simulink model "sample_model"  (R2023a)
settings: Solver=ode5  StartTime=0.0  StopTime=Inf  FixedStep=0.0001  RelTol=1e-3
PostLoadFcn:
  | , if any(exist('dsrtsu_mdlpostloadfcn', 'file') ~= 0), dsrtsu_mdlpostloadfcn('Execute', bdroot); end,
InitFcn:
  | , if any(exist('rtifpga_mdlclblib', 'file') ~= 0), rtifpga_mdlclblib('Init', bdroot); end,
values from neighbouring files (symbols this model uses):
  alpha = 0    [freq_sweep.m]    (also in freq_sweep_continous.m; single_test.m)
  k_harmonics = 7    [freq_sweep.m]    (also in freq_sweep_continous.m; single_test.m)
libraries: rti1202lib_adc_class1 x3, rti1202lib_dac_class1 x2, simulink x2, rti1202lib_base x1
(part 1 of 2)
Description:
  | Standard RTI1202 template.
  | Supported MATLAB version:  R2023a.
settings Model: Tag=RTI1202  DSRTSU_INTERNAL_RTI_VER=620  DSRTSU_INTERNAL_RTI_TYPE=rti1202  RTICANMMDATA=struct('GeneralSetupData',struct('modelroot','C:\Users\VM-User\Desktop\MigrationScripts','generalsettings',struct('filesettings',struct('destfolder',struct('Name','RTICANMM_FILES','Check',1),'buildfolder',struct('Name','.','Check',1),'AbsDestfolder',struct('Name','C:\Users\VM-User\Desktop\MigrationScripts\RTICANMM_FILES'),'AbsBuildfolder',struct('Name','C:\Users\VM-User\Desktop\MigrationScripts'))),'options',struct('addpaths',1,'rmpaths',1,'addtrcexclusion',true,'cannavigator',struct('checkmonitoring',0),'show_usrtrc',0,'use_usrtrc',0),'advanced',struct('options',ones(1,100)),'MPSetup',{{}},'RTI',struct('Type','RTI1202','Ver','7.17','Date','02-Nov-2021'),'modelname','','block','untitled'))  DSRTSU_INTERNAL_RTIFPGA=200  DSRTSU_INTERNAL_RTISTBM_VER=23.1  Creator=akb110  LastModifiedBy=dionl
settings SolverCC: AlgebraicLoopSolver=TrustRegion
settings DataIOCC: ReturnWorkspaceOutputs=off
settings OptimizationCC: BlockReduction=off  OptimizeBlockIOStorage=off  BufferReuse=off  ReuseModelBlockBuffer=off  GlobalBufferReuse=off  ExpressionFolding=off  LocalBlockOutputs=off  OptimizeDataStoreBuffers=off  BusAssignmentInplaceUpdate=off
settings DebuggingCC: UnconnectedInputMsg=warning  UnconnectedOutputMsg=warning  UnconnectedLineMsg=warning  PregeneratedLibrarySubsystemCodeDiagnostic=none  ArithmeticOperatorsInVariantConditions=warning
settings HardwareCC: ProdBitPerPointer=32  ProdBitPerSizeT=32  ProdBitPerPtrDiffT=32  ProdLargestAtomicInteger=Integer  ProdEndianess=BigEndian  ProdWordSize=32  ProdLongLongMode=on  ProdHWDeviceType=Custom Processor->Custom  TargetIntDivRoundTo=Zero  TargetEndianess=BigEndian  TargetHWDeviceType=Custom Processor->Custom
settings ModelReferenceCC: EnableRefExpFcnMdlSchedulingChecks=on  EnableParallelModelReferenceBuilds=on  ParallelModelReferenceMATLABWorkerInit=Load Top Model
settings SFSimCC: SimUseLocalCustomCode=off  MATLABDynamicMemAlloc=off  CustomCodeUndefinedFunction=UseInterfaceOnly
settings RTWCC: Description=dSPACE DS1202 Hardware Platform  SystemTargetFile=rti1202.tlc  MakeCommand=make_rti  TemplateMakefile=rti1202.tmf  RTWUseLocalCustomCode=off  DLArmComputeVersion=19.05
settings CodeAppCC: StateflowObjectComments=on
settings STFCustomTargetCC: TargetLangStandard=C89/C90 (ANSI)  ParMdlRefBuildCompliant=on  ConcurrentExecutionCompliant=off  GRTInterface=off  UseToolchainInfoCompliant=off  SystemTargetFile=rti1202.tlc
settings GRTTargetCC: TargetLangStandard=C89/C90 (ANSI)  CompOptLevelCompliant=off  ConcurrentExecutionCompliant=off  CombineOutputUpdateFcns=off  MatFileLogging=off  CPPClassGenCompliant=off  UseToolchainInfoCompliant=off
settings ConfigComp: CovMetricSettings=dswe

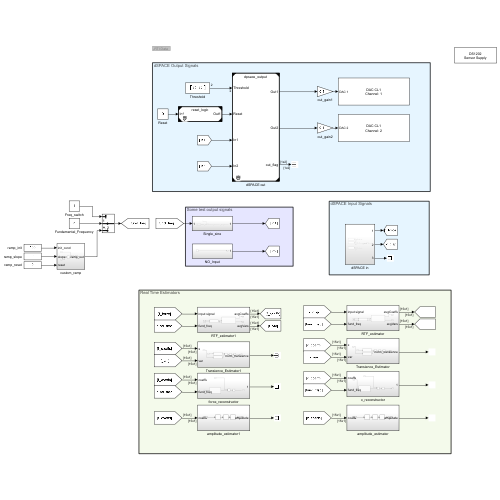
[thumbnail: Simulink's stored preview of the top-level diagram]
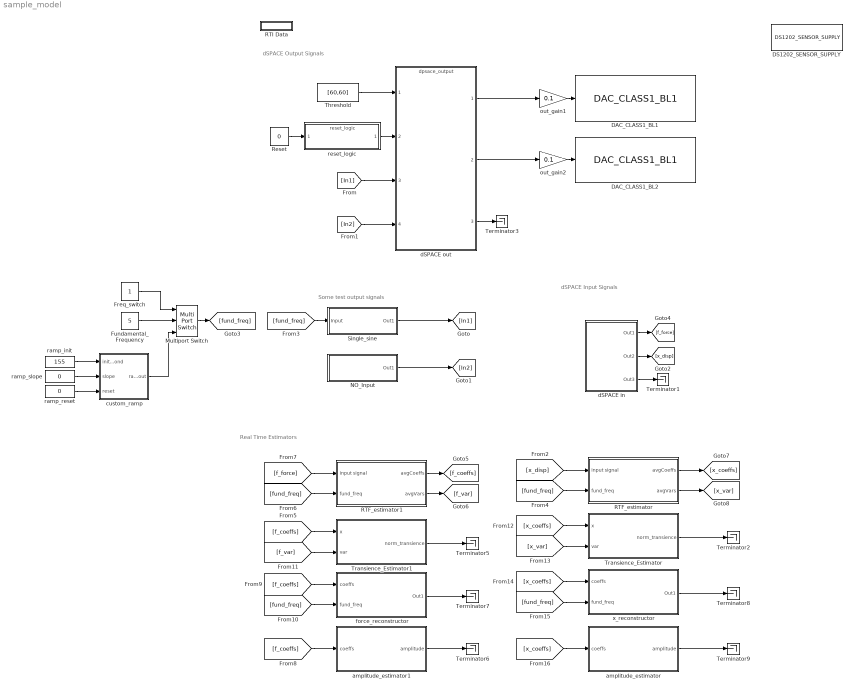
== system sample_model ==
  note: Real Time Estimators
  note: dSPACE Input Signals
  note: dSPACE Output Signals
  note: Some test output signals
  DAC_CLASS1_BL1 : rti1202lib_dac_class1/DAC_CLASS1_BL1  DSProperties=struct('RTI',struct('Version',uint32(2),'BlockType',struct('isSLSource',uint8(0),'isSLSink',uint8(1),'isHWSource',uint8(0),'isHWSink',uint8(1),'isSetup',uint8(0),'isInline',uint8(1),'isNonInline',uint8(0),'isInterrupt',uint8(0),'isChannelwise',uint8(1)),'IOBoardType',{{'DS120X','STD','DACC1'}},'UnitType','DAC','Identifier','DAC','DialogType','ML','BlockSet','NONE','SlaveProcessor','NONE'))  RTIBlockInterface=struct('InputPortsActive',1,'InputPortsWidth',int32(1),'InputPortsDataType',{{'SS_DOUBLE'}},'InputPortsName',{{['DAC 1']}},'DialogFcn','rti120xstddacc1dacgui','InitLevel',3,'IconTransparency','on','BlockDisplay',{{['DAC CL1\nChannel: 1'],'center'}},'BlockName',struct('Token',{{'DAC_CLASS1_BL1'}}))  RTIBlockParameters=struct('ChannelNo',{{1,'OFF',[]}},'ChannelNumOf',{{1,'OFF',[]}},'InitialValue1',{{0,'OFF',[-10 10]}},'InitialValue2',{{0,'OFF',[-10 10]}},'InitialValue3',{{0,'OFF',[-10 10]}},'InitialValue4',{{0,'OFF',[-10 10]}},'InitialValue5',{{0,'OFF',[-10 10]}},'InitialValue6',{{0,'OFF',[-10 10]}},'InitialValue7',{{0,'OFF',[-10 10]}},'InitialValue8',{{0,'OFF',[-10 10]}},'InitialValue9',{{0,'OFF',[-10 10]}},'InitialValue10',{{0,'OFF',[-10 10]}},'InitialValue11',{{0,'OFF',[-10 10]}},'InitialValue12',{{0,'OFF',[-10 10]}},'InitialValue13',{{0,'OFF',[-10 10]}},'InitialValue14',{{0,'OFF',[-10 10]}},'InitialValue15',{{0,'OFF',[-10 10]}},'InitialValue16',{{0,'OFF',[-10 10]}},'OutputMode',{{ones(1,16),'OFF',[1 2]}},'TermValue1',{{0,'OFF',[-10 10]}},'TermValue2',{{0,'OFF',[-10 10]}},'TermValue3',{{0,'OFF',[-10 10]}},'TermValue4',{{0,'OFF',[-10 10]}},'TermValue5',{{0,'OFF',[-10 10]}},'TermValue6',{{0,'OFF',[-10 10]}},'TermValue7',{{0,'OFF',[-10 10]}},'TermValue8',{{0,'OFF',[-10 10]}},'TermValue9',{{0,'OFF',[-10 10]}},'TermValue10',{{0,'OFF',[-10 10]}},'TermValue11',{{0,'OFF',[-10 10]}},'TermValue12',{{0,'OFF',[-10 10]}},'TermValue13',{{0,'OFF',[-10 10]}},'TermValue14',{{0,'OFF',[-10 10]}},'TermValue15',{{0,'OFF',[-10 10]}},'TermValue16',{{0,'OFF',[-10 10]}},'EnableTermMode',{{0,'OFF',[0 1]}},'TLCFileName',{{'rti120xdac_c1_dac','OFF',[]}},'InitialValueBuildCheck1',{{0,'OFF',[]}},'InitialValueBuildCheck2',{{0,'OFF',[]}},'InitialValueBuildCheck3',{{0,'OFF',[]}},'InitialValueBuildCheck4',{{0,'OFF',[]}},'InitialValueBuildCheck5',{{0,'OFF',[]}},'InitialValueBuildCheck6',{{0,'OFF',[]}},'InitialValueBuildCheck7',{{0,'OFF',[]}},'InitialValueBuildCheck8',{{0,'OFF',[]}},'InitialValueBuildCheck9',{{0,'OFF',[]}},'InitialValueBuildCheck10',{{0,'OFF',[]}},'InitialValueBuildCheck11',{{0,'OFF',[]}},'InitialValueBuildCheck12',{{0,'OFF',[]}},'InitialValueBuildCheck13',{{0,'OFF',[]}},'InitialValueBuildCheck14',{{0,'OFF',[]}},'InitialValueBuildCheck15',{{0,'OFF',[]}},'InitialValueBuildCheck16',{{0,'OFF',[]}},'TermValueBuildCheck1',{{0,'OFF',[]}},'TermValueBuildCheck2',{{0,'OFF',[]}},'TermValueBuildCheck3',{{0,'OFF',[]}},'TermValueBuildCheck4',{{0,'OFF',[]}},'TermValueBuildCheck5',{{0,'OFF',[]}},'TermValueBuildCheck6',{{0,'OFF',[]}},'TermValueBuildCheck7',{{0,'OFF',[]}},'TermValueBuildCheck8',{{0,'OFF',[]}},'TermValueBuildCheck9',{{0,'OFF',[]}},'TermValueBuildCheck10',{{0,'OFF',[]}},'TermValueBuildCheck11',{{0,'OFF',[]}},'TermValueBuildCheck12',{{0,'OFF',[]}},'TermValueBuildCheck13',{{0,'OFF',[]}},'TermValueBuildCheck14',{{0,'OFF',[]}},'TermValueBuildCheck15',{{0,'OFF',[]}},'TermValueBuildCheck16',{{0,'OFF',[]}})  RTISFcnParameters=struct('ChannelNo','int16','ChannelNumOf','int16','InitialValue1','double','InitialValue2','double','InitialValue3','double','InitialValue4','double','InitialValue5','double','InitialValue6','double','InitialValue7','double','InitialValue8','double','InitialValue9','double','InitialValue10','double','InitialValue11','double','InitialValue12','double','InitialValue13','double','InitialValue14','double','InitialValue15','double','InitialValue16','double','OutputMode','int16','TermValue1','double','TermValue2','double','TermValue3','double','TermValue4','double','TermValue5','double','TermValue6','double','TermValue7','double','TermValue8','double','TermValue9','double','TermValue10','double','TermValue11','double','TermValue12','double','TermValue13','double','TermValue14','double','TermValue15','double','TermValue16','double','EnableTermMode','int16','TLCFileName','char')  RTIBlockParaDefault=struct('ChannelNo',1,'ChannelNumOf',1,'InitialValue1',0,'InitialValue2',0,'InitialValue3',0,'InitialValue4',0,'InitialValue5',0,'InitialValue6',0,'InitialValue7',0,'InitialValue8',0,'InitialValue9',0,'InitialValue10',0,'InitialValue11',0,'InitialValue12',0,'InitialValue13',0,'InitialValue14',0,'InitialValue15',0,'InitialValue16',0,'OutputMode',ones(1,16),'TermValue1',0,'TermValue2',0,'TermValue3',0,'TermValue4',0,'TermValue5',0,'TermValue6',0,'TermValue7',0,'TermValue8',0,'TermValue9',0,'TermValue10',0,'TermValue11',0,'TermValue12',0,'TermValue13',0,'TermValue14',0,'TermValue15',0,'TermValue16',0,'EnableTermMode',0,'TLCFileName','rti120xdac_c1_dac','InitialValueBuildCheck1',0,'InitialValueBuildCheck2',0,'InitialValueBuildCheck3',0,'InitialValueBuildCheck4',0,'InitialValueBuildCheck5',0,'InitialValueBuildCheck6',0,'InitialValueBuildCheck7',0,'InitialValueBuildCheck8',0,'InitialValueBuildCheck9',0,'InitialValueBuildCheck10',0,'InitialValueBuildCheck11',0,'InitialValueBuildCheck12',0,'InitialValueBuildCheck13',0,'InitialValueBuildCheck14',0,'InitialValueBuildCheck15',0,'InitialValueBuildCheck16',0,'TermValueBuildCheck1',0,'TermValueBuildCheck2',0,'TermValueBuildCheck3',0,'TermValueBuildCheck4',0,'TermValueBuildCheck5',0,'TermValueBuildCheck6',0,'TermValueBuildCheck7',0,'TermValueBuildCheck8',0,'TermValueBuildCheck9',0,'TermValueBuildCheck10',0,'TermValueBuildCheck11',0,'TermValueBuildCheck12',0,'TermValueBuildCheck13',0,'TermValueBuildCheck14',0,'TermValueBuildCheck15',0,'TermValueBuildCheck16',0)
  DAC_CLASS1_BL2 : rti1202lib_dac_class1/DAC_CLASS1_BL1  DSProperties=struct('RTI',struct('Version',uint32(2),'BlockType',struct('isSLSource',uint8(0),'isSLSink',uint8(1),'isHWSource',uint8(0),'isHWSink',uint8(1),'isSetup',uint8(0),'isInline',uint8(1),'isNonInline',uint8(0),'isInterrupt',uint8(0),'isChannelwise',uint8(1)),'IOBoardType',{{'DS120X','STD','DACC1'}},'UnitType','DAC','Identifier','DAC','DialogType','ML','BlockSet','NONE','SlaveProcessor','NONE'))  RTIBlockInterface=struct('InputPortsActive',1,'InputPortsWidth',int32(1),'InputPortsDataType',{{'SS_DOUBLE'}},'InputPortsName',{{['DAC 2']}},'DialogFcn','rti120xstddacc1dacgui','InitLevel',3,'IconTransparency','on','BlockDisplay',{{['DAC CL1\nChannel: 2'],'center'}},'BlockName',struct('Token',{{'DAC_CLASS1_BL1'}}))  RTIBlockParameters=struct('ChannelNo',{{2,'OFF',[]}},'ChannelNumOf',{{1,'OFF',[]}},'InitialValue1',{{'0','OFF',[-10 10]}},'InitialValue2',{{'0','OFF',[-10 10]}},'InitialValue3',{{'0','OFF',[-10 10]}},'InitialValue4',{{'0','OFF',[-10 10]}},'InitialValue5',{{'0','OFF',[-10 10]}},'InitialValue6',{{'0','OFF',[-10 10]}},'InitialValue7',{{'0','OFF',[-10 10]}},'InitialValue8',{{'0','OFF',[-10 10]}},'InitialValue9',{{'0','OFF',[-10 10]}},'InitialValue10',{{'0','OFF',[-10 10]}},'InitialValue11',{{'0','OFF',[-10 10]}},'InitialValue12',{{'0','OFF',[-10 10]}},'InitialValue13',{{'0','OFF',[-10 10]}},'InitialValue14',{{'0','OFF',[-10 10]}},'InitialValue15',{{'0','OFF',[-10 10]}},'InitialValue16',{{'0','OFF',[-10 10]}},'OutputMode',{{ones(1,16),'OFF',[1 2]}},'TermValue1',{{'0','OFF',[-10 10]}},'TermValue2',{{'0','OFF',[-10 10]}},'TermValue3',{{'0','OFF',[-10 10]}},'TermValue4',{{'0','OFF',[-10 10]}},'TermValue5',{{'0','OFF',[-10 10]}},'TermValue6',{{'0','OFF',[-10 10]}},'TermValue7',{{'0','OFF',[-10 10]}},'TermValue8',{{'0','OFF',[-10 10]}},'TermValue9',{{'0','OFF',[-10 10]}},'TermValue10',{{'0','OFF',[-10 10]}},'TermValue11',{{'0','OFF',[-10 10]}},'TermValue12',{{'0','OFF',[-10 10]}},'TermValue13',{{'0','OFF',[-10 10]}},'TermValue14',{{'0','OFF',[-10 10]}},'TermValue15',{{'0','OFF',[-10 10]}},'TermValue16',{{'0','OFF',[-10 10]}},'EnableTermMode',{{0,'OFF',[0 1]}},'TLCFileName',{{'rti120xdac_c1_dac','OFF',[]}},'InitialValueBuildCheck1',{{0,'OFF',[]}},'InitialValueBuildCheck2',{{1,'OFF',[]}},'InitialValueBuildCheck3',{{0,'OFF',[]}},'InitialValueBuildCheck4',{{0,'OFF',[]}},'InitialValueBuildCheck5',{{0,'OFF',[]}},'InitialValueBuildCheck6',{{0,'OFF',[]}},'InitialValueBuildCheck7',{{0,'OFF',[]}},'InitialValueBuildCheck8',{{0,'OFF',[]}},'InitialValueBuildCheck9',{{0,'OFF',[]}},'InitialValueBuildCheck10',{{0,'OFF',[]}},'InitialValueBuildCheck11',{{0,'OFF',[]}},'InitialValueBuildCheck12',{{0,'OFF',[]}},'InitialValueBuildCheck13',{{0,'OFF',[]}},'InitialValueBuildCheck14',{{0,'OFF',[]}},'InitialValueBuildCheck15',{{0,'OFF',[]}},'InitialValueBuildCheck16',{{0,'OFF',[]}},'TermValueBuildCheck1',{{0,'OFF',[]}},'TermValueBuildCheck2',{{0,'OFF',[]}},'TermValueBuildCheck3',{{0,'OFF',[]}},'TermValueBuildCheck4',{{0,'OFF',[]}},'TermValueBuildCheck5',{{0,'OFF',[]}},'TermValueBuildCheck6',{{0,'OFF',[]}},'TermValueBuildCheck7',{{0,'OFF',[]}},'TermValueBuildCheck8',{{0,'OFF',[]}},'TermValueBuildCheck9',{{0,'OFF',[]}},'TermValueBuildCheck10',{{0,'OFF',[]}},'TermValueBuildCheck11',{{0,'OFF',[]}},'TermValueBuildCheck12',{{0,'OFF',[]}},'TermValueBuildCheck13',{{0,'OFF',[]}},'TermValueBuildCheck14',{{0,'OFF',[]}},'TermValueBuildCheck15',{{0,'OFF',[]}},'TermValueBuildCheck16',{{0,'OFF',[]}})  RTISFcnParameters=struct('ChannelNo','int16','ChannelNumOf','int16','InitialValue1','double','InitialValue2','double','InitialValue3','double','InitialValue4','double','InitialValue5','double','InitialValue6','double','InitialValue7','double','InitialValue8','double','InitialValue9','double','InitialValue10','double','InitialValue11','double','InitialValue12','double','InitialValue13','double','InitialValue14','double','InitialValue15','double','InitialValue16','double','OutputMode','int16','TermValue1','double','TermValue2','double','TermValue3','double','TermValue4','double','TermValue5','double','TermValue6','double','TermValue7','double','TermValue8','double','TermValue9','double','TermValue10','double','TermValue11','double','TermValue12','double','TermValue13','double','TermValue14','double','TermValue15','double','TermValue16','double','EnableTermMode','int16','TLCFileName','char')  RTIBlockParaDefault=struct('ChannelNo',1,'ChannelNumOf',1,'InitialValue1',0,'InitialValue2',0,'InitialValue3',0,'InitialValue4',0,'InitialValue5',0,'InitialValue6',0,'InitialValue7',0,'InitialValue8',0,'InitialValue9',0,'InitialValue10',0,'InitialValue11',0,'InitialValue12',0,'InitialValue13',0,'InitialValue14',0,'InitialValue15',0,'InitialValue16',0,'OutputMode',ones(1,16),'TermValue1',0,'TermValue2',0,'TermValue3',0,'TermValue4',0,'TermValue5',0,'TermValue6',0,'TermValue7',0,'TermValue8',0,'TermValue9',0,'TermValue10',0,'TermValue11',0,'TermValue12',0,'TermValue13',0,'TermValue14',0,'TermValue15',0,'TermValue16',0,'EnableTermMode',0,'TLCFileName','rti120xdac_c1_dac','InitialValueBuildCheck1',0,'InitialValueBuildCheck2',0,'InitialValueBuildCheck3',0,'InitialValueBuildCheck4',0,'InitialValueBuildCheck5',0,'InitialValueBuildCheck6',0,'InitialValueBuildCheck7',0,'InitialValueBuildCheck8',0,'InitialValueBuildCheck9',0,'InitialValueBuildCheck10',0,'InitialValueBuildCheck11',0,'InitialValueBuildCheck12',0,'InitialValueBuildCheck13',0,'InitialValueBuildCheck14',0,'InitialValueBuildCheck15',0,'InitialValueBuildCheck16',0,'TermValueBuildCheck1',0,'TermValueBuildCheck2',0,'TermValueBuildCheck3',0,'TermValueBuildCheck4',0,'TermValueBuildCheck5',0,'TermValueBuildCheck6',0,'TermValueBuildCheck7',0,'TermValueBuildCheck8',0,'TermValueBuildCheck9',0,'TermValueBuildCheck10',0,'TermValueBuildCheck11',0,'TermValueBuildCheck12',0,'TermValueBuildCheck13',0,'TermValueBuildCheck14',0,'TermValueBuildCheck15',0,'TermValueBuildCheck16',0)
  DS1202_SENSOR_SUPPLY : rti1202lib_base/DS1202_SENSOR_SUPPLY  DSProperties=struct('RTI',struct('Version',uint32(1),'BlockType',struct('isSLSource',uint8(0),'isSLSink',uint8(0),'isHWSource',uint8(0),'isHWSink',uint8(1),'isSetup',uint8(0),'isInline',uint8(1),'isNonInline',uint8(0),'isInterrupt',uint8(0),'isChannelwise',uint8(0)),'IOBoardType',{{'DS120X','BASE'}},'UnitType','SENSORSUPPLY','Identifier','SENSORSUPPLY','DialogType','ML','BlockSet','NONE','SlaveProcessor','NONE'))  RTIBlockInterface=struct('OutputPortsActive',0,'OutputPortsWidth',int32(0),'DialogFcn','rti120xbasesensorsupplygui','InitLevel',3,'IconTransparency','off','BlockDisplay',{{['DS1202\nSensor Supply'],'center'}},'BlockName',struct('Token',{{'DS1202_SENSOR_SUPPLY'}}))  RTIBlockParameters=struct('Voltage',{{'14','OFF',[2 20]}},'TLCFileName',{{'rti120xbase_sensor_supply','OFF',[]}})  RTISFcnParameters=struct('Voltage','double','TLCFileName','char')  RTIBlockParaDefault=struct('Voltage',2,'TLCFileName','rti120xbase_sensor_supply')
  Freq_switch : Constant
  Fundamental_Frequency : Constant  Value=5
  Multiport Switch : MultiPortSwitch  Inputs=2  SaturateOnIntegerOverflow=off  InputSameDT=off
  NO_Input : Subsystem
  RTF_estimator : Subsystem
  RTF_estimator1 : Subsystem
  RTI Data : Subsystem  Tag=struct('RTIDataServer',struct('RTIDataServerVs','2','RTIModelDescription','struct(''main'',''sample_model'',''sub'','''',''isMp'',0)'))  LoadFcn="if exist('rtidc'), try,  rtidc('DataHostBlockClbLoad', gcbh); catch, disp(['Warning: ''LoadFcn'' for RTI Data block failed: ' lasterr]); end, end,"  mask(RTI_DATA_HOST){}
      mask help:
      | RTI Data Block.
      | This block is used by RTI to store internal model-dependent data.
      | Please keep this block on the root level of the model. Deleting this block will result in data loss.
      |
      | NEVER DELETE OR COPY THIS BLOCK!
      settings: CopyFcn="if exist('rtidc'), try,  rtidc('DataHostBlockClbCopy', gcbh); catch, disp(['Warning: ''CopyFcn'' for RTI Data block failed: ' lasterr]); end, end,"  DeleteFcn="if exist('rtidc'), try,  rtidc('DataHostBlockClbDelete', gcbh); catch, disp(['Warning: ''DeleteFcn'' for RTI Data block failed: ' lasterr]); end, end,"  ModelCloseFcn="if exist('rtidc'), try,  rtidc('DataHostBlockClbModelClose', gcbh); catch, disp(['Warning: ''ModelCloseFcn'' for RTI Data block failed: ' lasterr]); end, end,"  PreSaveFcn="if exist('rtidc'), try,  rtidc('DataHostBlockClbPreSave', gcbh); catch, disp(['Warning: ''PreSaveFcn'' for RTI Data block failed: ' lasterr]); end, end,"  PostSaveFcn="if exist('rtidc'), try,  rtidc('DataHostBlockClbPostSave', gcbh); catch, disp(['Warning: ''PostSaveFcn'' for RTI Data block failed: ' lasterr]); end, end,"  NameChangeFcn="if exist('rtidc'), try,  rtidc('DataHostBlockClbNameChange', gcbh); catch, disp(['Warning: ''NameChangeFcn'' for RTI Data block failed: ' lasterr]); end, end,"
      mask Help:
      | RTI Data Block.
      | This block is used by RTI to store internal model-dependent data.
      | Please keep this block on the root level of the model. Deleting this block will result in data loss.
      | 
      | NEVER DELETE OR COPY THIS BLOCK!
      mask Display:
      | text(0.5, 0.5, 'RTI Data', 'HorizontalAlignment', 'center');
      | plot([1 0]);
  Reset : Constant  Value=0
  Single_sine : Subsystem
  Terminator{1..3,5..9} (8 alike) : Terminator
  Threshold : Constant  Value=[60,60]
  Transience_Estimator : Subsystem
  Transience_Estimator1 : Subsystem
  amplitude_estimator : Subsystem
  amplitude_estimator1 : Subsystem
  custom_ramp : Subsystem
  dSPACE in : Subsystem
  dSPACE out : ModelReference  ModelNameDialog=dpsace_output.slxp  ModelReferenceVersion=1.2  CopyOfModelProtected=on
  force_reconstructor : Subsystem
  out_gain1 : Gain  Gain=0.1
  out_gain2 : Gain  Gain=0.1
  ramp_init : Constant  Value=155
  ramp_reset : Constant  Value=0
  ramp_slope : Constant  Value=0
  reset_logic : ModelReference  ModelNameDialog=reset_logic.slxp  ModelReferenceVersion=1.2  CopyOfModelProtected=on
  x_reconstructor : Subsystem
  wires:
  out_gain1/1 -> DAC_CLASS1_BL1/1
  Single_sine/1(Out1) -> [In1]
  NO_Input/1(Out1) -> [In2]
  [In2] -> dSPACE out/4
  [In1] -> dSPACE out/3
  Threshold/1 -> dSPACE out/1
  dSPACE out/1 -> out_gain1/1
  dSPACE out/2 -> out_gain2/1
  reset_logic/1 -> dSPACE out/2
  Reset/1 -> reset_logic/1
  out_gain2/1 -> DAC_CLASS1_BL2/1
  dSPACE out/3 -> Terminator3/1
  dSPACE in/1(Out1) -> [f_force]
  dSPACE in/2(Out2) -> [x_disp]
  dSPACE in/3(Out3) -> Terminator1/1
  [x_disp] -> RTF_estimator/1(input signal)
  [fund_freq] -> RTF_estimator/2(fund_freq)
  Fundamental_Frequency/1 -> Multiport Switch/2
  [fund_freq] -> Single_sine/1(Input)
  Multiport Switch/1 -> [fund_freq]
  custom_ramp/1(ramp_out) -> Multiport Switch/3
  amplitude_estimator1/1(amplitude) -> Terminator6/1
  Transience_Estimator1/1(norm_transience) -> Terminator5/1
  [fund_freq] -> RTF_estimator1/2(fund_freq)
  [f_force] -> RTF_estimator1/1(input signal)
  force_reconstructor/1(Out1) -> Terminator7/1
  RTF_estimator1/1(avgCoeffs) -> [f_coeffs]
  [f_coeffs] -> Transience_Estimator1/1(x)
  [f_coeffs] -> amplitude_estimator1/1(coeffs)
  [f_coeffs] -> force_reconstructor/1(coeffs)
  [fund_freq] -> force_reconstructor/2(fund_freq)
  RTF_estimator1/2(avgVars) -> [f_var]
  [f_var] -> Transience_Estimator1/2(var)
  RTF_estimator/1(avgCoeffs) -> [x_coeffs]
  RTF_estimator/2(avgVars) -> [x_var]
  [x_coeffs] -> Transience_Estimator/1(x)
  [x_var] -> Transience_Estimator/2(var)
  Transience_Estimator/1(norm_transience) -> Terminator2/1
  [x_coeffs] -> x_reconstructor/1(coeffs)
  [fund_freq] -> x_reconstructor/2(fund_freq)
  [x_coeffs] -> amplitude_estimator/1(coeffs)
  amplitude_estimator/1(amplitude) -> Terminator9/1
  x_reconstructor/1(Out1) -> Terminator8/1
  Freq_switch/1 -> Multiport Switch/1
  ramp_init/1 -> custom_ramp/1(init_cond)
  ramp_slope/1 -> custom_ramp/2(slope)
  ramp_reset/1 -> custom_ramp/3(reset)

== system sample_model/NO_Input ==
  N/A : Constant  Value=0
  Out1 : Outport
  wires:
  N/A/1 -> Out1/1

== system sample_model/RTF_estimator ==
  input signal : Inport
  fund_freq : Inport  Port=2
  MATLAB Function1 : MATLAB Function  TreatAsAtomicUnit=on
  Subsystem : Subsystem
  Terminator : Terminator
  avgCoeffs : Outport
  avgVars : Outport  Port=2
  wires:
  input signal/1 -> Subsystem/1(input signal)
  Subsystem/2(Phase1) -> Terminator/1
  fund_freq/1 -> Subsystem/2(fund_freq)
  Subsystem/1(Fourier1) -> MATLAB Function1/1(Coeffs)
  MATLAB Function1/2(varCoeffs) -> avgVars/1
  MATLAB Function1/1(avgCoeffs) -> avgCoeffs/1  "Fourier"

== system sample_model/RTF_estimator1 ==
  input signal : Inport
  fund_freq : Inport  Port=2
  MATLAB Function1 : MATLAB Function  TreatAsAtomicUnit=on
  Subsystem : Subsystem
  Terminator : Terminator
  avgCoeffs : Outport
  avgVars : Outport  Port=2
  wires:
  MATLAB Function1/1(avgCoeffs) -> avgCoeffs/1  "Fourier"
  MATLAB Function1/2(varCoeffs) -> avgVars/1
  Subsystem/1(Fourier1) -> MATLAB Function1/1(Coeffs)
  fund_freq/1 -> Subsystem/2(fund_freq)
  Subsystem/2(Phase1) -> Terminator/1
  input signal/1 -> Subsystem/1(input signal)

== system sample_model/RTI Data ==
  RTI Data Store : Subsystem  Tag="struct('public',struct('sub',struct('name',{{'sample_model'}},'data',{{struct('TH',struct('thTaskInfo',struct('taskType',{'TIMER','HWINT','TMRINT','SWINT','GLINT'},'tasksNumOf',{1,0,0,0,0},'srcIds',{{'TIMERA'},{},{},{},{}},'taskNames',{{['Timer Task 1']},{},{},{},{}})),'th_tc',struct('dataType','TASK','taskGroupId','','taskGroupList',{{}},'taskSchedulingPolicy','FCFS','taskType','TIMER','blkh',-1,'srcId','TIMERA','srcSgnName',['Timer A interrupt'],'srcCpuName','','taskName',['Timer Task 1  [0.0001] s'],'taskNameDisplayExt','','smplTime',0.0001,'smplTimeOffs',0,'hasFixedPriority',0,'priority',1,'hasFixedOvc',0,'ovcType',1,'ovcMax',1),'tc_th',struct('dataType','TASK','taskGroupId','','taskGroupList',{{}},'taskSchedulingPolicy','FCFS','taskType','TIMER','blkh',-1,'srcId','TIMERA','srcSgnName',['Timer A interrupt'],'srcCpuName','','taskName',['Timer Task 1  [0.0001] s'],'taskNameDisplayExt','','smplTime',0.0001,'smplTimeOffs',0,'hasFixedPriority',0,'priority',1,'hasFixedOvc',0,'ovcType',1,'ovcMax',1))}})),'private',struct('version',struct('dsVer',uint32(2)),'access',struct('modified',['18-Jul-2025 17:09:18'],'type','Model','isPerm',1)))"  mask(RTI_DATA_STORE){}
      mask help:
      | RTI Data Store Block. This block is used by RTI to store internal model dependent data. Deleting this block will result in data loss.
      |
      | NEVER DELETE, COPY, OR MODIFY THIS BLOCK!
      mask Help:
      | RTI Data Store Block. This block is used by RTI to store internal model dependent data. Deleting this block will result in data loss.
      | 
      | NEVER DELETE, COPY, OR MODIFY THIS BLOCK!
      mask Display: text(0.5, 0.5, ' ', 'HorizontalAlignment', 'center');

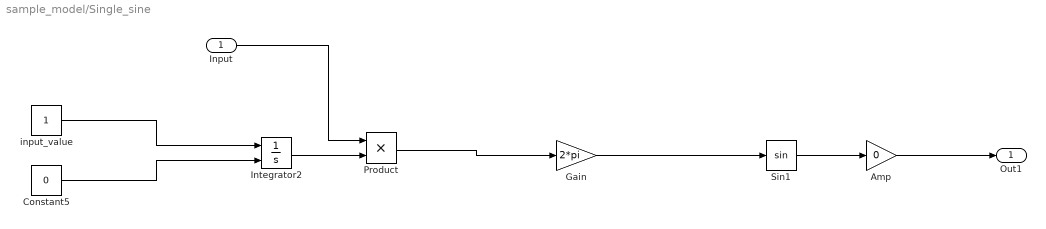
== system sample_model/Single_sine ==
  Input : Inport
  Amp : Gain  Gain=0
  Constant5 : Constant  Value=0
  Gain : Gain  Gain=2*pi
  Integrator2 : Integrator  ExternalReset=rising
  Product : Product
  Sin1 : Trigonometry
  input_value : Constant
  Out1 : Outport
  wires:
  input_value/1 -> Integrator2/1
  Product/1 -> Gain/1
  Gain/1 -> Sin1/1
  Amp/1 -> Out1/1
  Integrator2/1 -> Product/2
  Sin1/1 -> Amp/1
  Constant5/1 -> Integrator2/2
  Input/1 -> Product/1

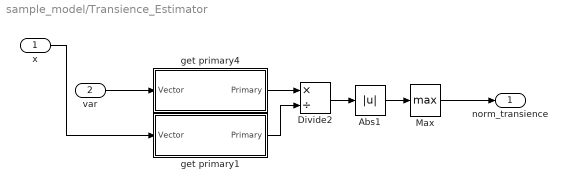
== system sample_model/Transience_Estimator ==
  x : Inport
  var : Inport  Port=2
  Abs1 : Abs  SaturateOnIntegerOverflow=off
  Divide2 : Product  Inputs=*/
  Max : MinMax  Function=max
  get primary1 : Subsystem
  get primary4 : Subsystem
  norm_transience : Outport
  wires:
  Divide2/1 -> Abs1/1
  x/1 -> get primary1/1(Vector)
  get primary1/1(Primary) -> Divide2/2
  get primary4/1(Primary) -> Divide2/1
  var/1 -> get primary4/1(Vector)
  Abs1/1 -> Max/1
  Max/1 -> norm_transience/1

== system sample_model/Transience_Estimator1 ==
  x : Inport
  var : Inport  Port=2
  Abs1 : Abs  SaturateOnIntegerOverflow=off
  Divide2 : Product  Inputs=*/
  Max : MinMax  Function=max
  get primary1 : Subsystem
  get primary4 : Subsystem
  norm_transience : Outport
  wires:
  Max/1 -> norm_transience/1
  Abs1/1 -> Max/1
  var/1 -> get primary4/1(Vector)
  get primary4/1(Primary) -> Divide2/1
  get primary1/1(Primary) -> Divide2/2
  x/1 -> get primary1/1(Vector)
  Divide2/1 -> Abs1/1

== system sample_model/amplitude_estimator ==
  coeffs : Inport
  Sqrt : Sqrt
  Square : Math  Operator=square
  Sum of Elements : Sum  Inputs=+
  amplitude : Outport
  wires:
  Sum of Elements/1 -> Sqrt/1
  Square/1 -> Sum of Elements/1
  coeffs/1 -> Square/1
  Sqrt/1 -> amplitude/1

== system sample_model/amplitude_estimator1 ==
  coeffs : Inport
  Sqrt : Sqrt
  Square : Math  Operator=square
  Sum of Elements : Sum  Inputs=+
  amplitude : Outport
  wires:
  Sqrt/1 -> amplitude/1
  coeffs/1 -> Square/1
  Square/1 -> Sum of Elements/1
  Sum of Elements/1 -> Sqrt/1

== system sample_model/custom_ramp ==
  init_cond : Inport
  slope : Inport  Port=2
  reset : Inport  Port=3
  Add : Sum
  Integrator : Integrator  ExternalReset=either
  Saturation : Saturate  UpperLimit=180  LowerLimit=155
  ramp_out : Outport
  wires:
  init_cond/1 -> Add/1
  Integrator/1 -> Add/2
  Saturation/1 -> ramp_out/1
  reset/1 -> Integrator/2
  Add/1 -> Saturation/1
  slope/1 -> Integrator/1

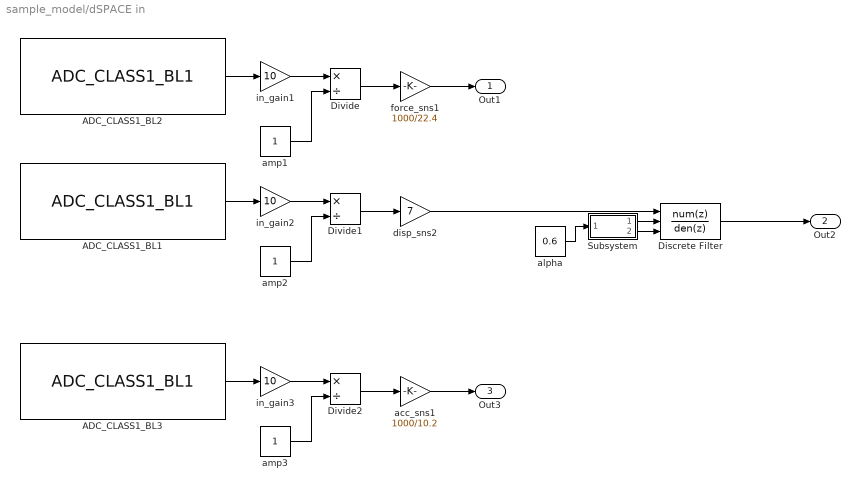
== system sample_model/dSPACE in ==
  ADC_CLASS1_BL1 : rti1202lib_adc_class1/ADC_CLASS1_BL1  DSProperties=struct('RTI',struct('Version',uint32(1),'BlockType',struct('isSLSource',uint8(1),'isSLSink',uint8(1),'isHWSource',uint8(0),'isHWSink',uint8(1),'isSetup',uint8(0),'isInline',uint8(1),'isNonInline',uint8(0),'isInterrupt',uint8(0),'isChannelwise',uint8(1)),'IOBoardType',{{'DS120X','STD','ADCC1'}},'UnitType','ADC','Identifier','ADC','DialogType','ML','BlockSet','NONE','SlaveProcessor','NONE'))  RTIBlockInterface=struct('InputPortsActive',0,'InputPortsWidth',int32(1),'InputPortsDataType',{{'SS_BOOLEAN'}},'InputPortsName',{{'Continue'}},'OutputPortsActive',[1 0],'OutputPortsWidth',int32([1 1]),'OutputPortsDataType',{{'SS_DOUBLE','SS_INT16'}},'OutputPortsName',{{'ADC','Status'}},'DialogFcn','rti120xstdadcc1adcgui','SampleTime',{{-1}},'InitLevel',3,'IconTransparency','on','BlockDisplay',{{['ADC CL1\nChannel: 3'],'center'}},'BlockName',struct('Token',{{'ADC_CLASS1_BL1'}}))  RTIBlockParameters=struct('ReadMode',{{1,'OFF',[1 2]}},'ChannelNo',{{3,'OFF',[]}},'ConversionMode',{{1,'OFF',[1 2]}},'TriggerSource',{{1,'OFF',[1 2]}},'TriggerLineIn',{{1,'OFF',[1 16]}},'SampleMode',{{1,'OFF',[1 2]}},'BurstTriggerSource',{{1,'OFF',[1 2]}},'BurstTriggerLine',{{1,'OFF',[1 16]}},'ConvTriggerSource',{{3,'OFF',[1 3]}},'ConvTriggerLine',{{1,'OFF',[1 16]}},'ConvPeriod',{{'100e-6','OFF',[1e-6 1.34]}},'ConvPeriodCheck',{{0,'OFF',[]}},'BurstSize',{{'10','OFF',[]}},'BurstSizeCheck',{{0,'OFF',[]}},'DataSetOffset',{{'0','OFF',[]}},'DataSetOffsetCheck',{{0,'OFF',[]}},'DataSetLength',{{'1','OFF',[]}},'DataSetLengthCheck',{{0,'OFF',[]}},'EnableTriggerEvent',{{0,'OFF',[0 1]}},'TriggerMode',{{2,'OFF',[1 3]}},'TriggerLineOut',{{1,'OFF',[1 16]}},'ADCSWStartEnable',{{0,'OFF',[0 1]}},'SampleTime',{{'-1','OFF',[-1 inf]}},'SampleTimeCheck',{{1,'OFF',[]}},'StatusPortEnable',{{0,'OFF',[0 1]}},'TLCFileName',{{'rti120xadc_c1_adc','OFF',[]}})  RTISFcnParameters=struct('ReadMode','int16','ChannelNo','int16','ConversionMode','int16','TriggerSource','int16','TriggerLineIn','int16','SampleMode','int16','BurstTriggerSource','int16','BurstTriggerLine','int16','ConvTriggerSource','int16','ConvTriggerLine','int16','ConvPeriod','double','BurstSize','int16','DataSetOffset','int16','DataSetLength','int16','EnableTriggerEvent','int16','TriggerMode','int16','TriggerLineOut','int16','ADCSWStartEnable','int16','SampleTime','double','StatusPortEnable','int16','TLCFileName','char')  RTIBlockParaDefault=struct('ReadMode',1,'ChannelNo',1,'ConversionMode',1,'TriggerSource',1,'TriggerLineIn',1,'SampleMode',1,'BurstTriggerSource',1,'BurstTriggerLine',1,'ConvTriggerSource',3,'ConvTriggerLine',1,'ConvPeriod',0.0001,'ConvPeriodCheck',0,'BurstSize',10,'BurstSizeCheck',0,'DataSetOffset',0,'DataSetOffsetCheck',0,'DataSetLength',1,'DataSetLengthCheck',0,'EnableTriggerEvent',0,'TriggerMode',2,'TriggerLineOut',1,'ADCSWStartEnable',0,'SampleTime',-1,'SampleTimeCheck',1,'StatusPortEnable',0,'TLCFileName','rti120xadc_c1_adc')
  ADC_CLASS1_BL2 : rti1202lib_adc_class1/ADC_CLASS1_BL1  DSProperties=struct('RTI',struct('Version',uint32(1),'BlockType',struct('isSLSource',uint8(1),'isSLSink',uint8(1),'isHWSource',uint8(0),'isHWSink',uint8(1),'isSetup',uint8(0),'isInline',uint8(1),'isNonInline',uint8(0),'isInterrupt',uint8(0),'isChannelwise',uint8(1)),'IOBoardType',{{'DS120X','STD','ADCC1'}},'UnitType','ADC','Identifier','ADC','DialogType','ML','BlockSet','NONE','SlaveProcessor','NONE'))  RTIBlockInterface=struct('InputPortsActive',0,'InputPortsWidth',int32(1),'InputPortsDataType',{{'SS_BOOLEAN'}},'InputPortsName',{{'Continue'}},'OutputPortsActive',[1 0],'OutputPortsWidth',int32([1 1]),'OutputPortsDataType',{{'SS_DOUBLE','SS_INT16'}},'OutputPortsName',{{'ADC','Status'}},'DialogFcn','rti120xstdadcc1adcgui','SampleTime',{{-1}},'InitLevel',3,'IconTransparency','on','BlockDisplay',{{['ADC CL1\nChannel: 1'],'center'}},'BlockName',struct('Token',{{'ADC_CLASS1_BL1'}}))  RTIBlockParameters=struct('ReadMode',{{1,'OFF',[1 2]}},'ChannelNo',{{1,'OFF',[]}},'ConversionMode',{{1,'OFF',[1 2]}},'TriggerSource',{{1,'OFF',[1 2]}},'TriggerLineIn',{{1,'OFF',[1 16]}},'SampleMode',{{1,'OFF',[1 2]}},'BurstTriggerSource',{{1,'OFF',[1 2]}},'BurstTriggerLine',{{1,'OFF',[1 16]}},'ConvTriggerSource',{{3,'OFF',[1 3]}},'ConvTriggerLine',{{1,'OFF',[1 16]}},'ConvPeriod',{{'100e-6','OFF',[1e-6 1.34]}},'ConvPeriodCheck',{{0,'OFF',[]}},'BurstSize',{{'10','OFF',[]}},'BurstSizeCheck',{{0,'OFF',[]}},'DataSetOffset',{{'0','OFF',[]}},'DataSetOffsetCheck',{{0,'OFF',[]}},'DataSetLength',{{'1','OFF',[]}},'DataSetLengthCheck',{{0,'OFF',[]}},'EnableTriggerEvent',{{0,'OFF',[0 1]}},'TriggerMode',{{2,'OFF',[1 3]}},'TriggerLineOut',{{1,'OFF',[1 16]}},'ADCSWStartEnable',{{0,'OFF',[0 1]}},'SampleTime',{{'-1','OFF',[-1 inf]}},'SampleTimeCheck',{{1,'OFF',[]}},'StatusPortEnable',{{0,'OFF',[0 1]}},'TLCFileName',{{'rti120xadc_c1_adc','OFF',[]}})  RTISFcnParameters=struct('ReadMode','int16','ChannelNo','int16','ConversionMode','int16','TriggerSource','int16','TriggerLineIn','int16','SampleMode','int16','BurstTriggerSource','int16','BurstTriggerLine','int16','ConvTriggerSource','int16','ConvTriggerLine','int16','ConvPeriod','double','BurstSize','int16','DataSetOffset','int16','DataSetLength','int16','EnableTriggerEvent','int16','TriggerMode','int16','TriggerLineOut','int16','ADCSWStartEnable','int16','SampleTime','double','StatusPortEnable','int16','TLCFileName','char')  RTIBlockParaDefault=struct('ReadMode',1,'ChannelNo',1,'ConversionMode',1,'TriggerSource',1,'TriggerLineIn',1,'SampleMode',1,'BurstTriggerSource',1,'BurstTriggerLine',1,'ConvTriggerSource',3,'ConvTriggerLine',1,'ConvPeriod',0.0001,'ConvPeriodCheck',0,'BurstSize',10,'BurstSizeCheck',0,'DataSetOffset',0,'DataSetOffsetCheck',0,'DataSetLength',1,'DataSetLengthCheck',0,'EnableTriggerEvent',0,'TriggerMode',2,'TriggerLineOut',1,'ADCSWStartEnable',0,'SampleTime',-1,'SampleTimeCheck',1,'StatusPortEnable',0,'TLCFileName','rti120xadc_c1_adc')
  ADC_CLASS1_BL3 : rti1202lib_adc_class1/ADC_CLASS1_BL1  DSProperties=struct('RTI',struct('Version',uint32(1),'BlockType',struct('isSLSource',uint8(1),'isSLSink',uint8(1),'isHWSource',uint8(0),'isHWSink',uint8(1),'isSetup',uint8(0),'isInline',uint8(1),'isNonInline',uint8(0),'isInterrupt',uint8(0),'isChannelwise',uint8(1)),'IOBoardType',{{'DS120X','STD','ADCC1'}},'UnitType','ADC','Identifier','ADC','DialogType','ML','BlockSet','NONE','SlaveProcessor','NONE'))  RTIBlockInterface=struct('InputPortsActive',0,'InputPortsWidth',int32(1),'InputPortsDataType',{{'SS_BOOLEAN'}},'InputPortsName',{{'Continue'}},'OutputPortsActive',[1 0],'OutputPortsWidth',int32([1 1]),'OutputPortsDataType',{{'SS_DOUBLE','SS_INT16'}},'OutputPortsName',{{'ADC','Status'}},'DialogFcn','rti120xstdadcc1adcgui','SampleTime',{{-1}},'InitLevel',3,'IconTransparency','on','BlockDisplay',{{['ADC CL1\nChannel: 2'],'center'}},'BlockName',struct('Token',{{'ADC_CLASS1_BL1'}}))  RTIBlockParameters=struct('ReadMode',{{1,'OFF',[1 2]}},'ChannelNo',{{2,'OFF',[]}},'ConversionMode',{{1,'OFF',[1 2]}},'TriggerSource',{{1,'OFF',[1 2]}},'TriggerLineIn',{{1,'OFF',[1 16]}},'SampleMode',{{1,'OFF',[1 2]}},'BurstTriggerSource',{{1,'OFF',[1 2]}},'BurstTriggerLine',{{1,'OFF',[1 16]}},'ConvTriggerSource',{{3,'OFF',[1 3]}},'ConvTriggerLine',{{1,'OFF',[1 16]}},'ConvPeriod',{{'100e-6','OFF',[1e-6 1.34]}},'ConvPeriodCheck',{{0,'OFF',[]}},'BurstSize',{{'10','OFF',[]}},'BurstSizeCheck',{{0,'OFF',[]}},'DataSetOffset',{{'0','OFF',[]}},'DataSetOffsetCheck',{{0,'OFF',[]}},'DataSetLength',{{'1','OFF',[]}},'DataSetLengthCheck',{{0,'OFF',[]}},'EnableTriggerEvent',{{0,'OFF',[0 1]}},'TriggerMode',{{2,'OFF',[1 3]}},'TriggerLineOut',{{1,'OFF',[1 16]}},'ADCSWStartEnable',{{0,'OFF',[0 1]}},'SampleTime',{{'-1','OFF',[-1 inf]}},'SampleTimeCheck',{{1,'OFF',[]}},'StatusPortEnable',{{0,'OFF',[0 1]}},'TLCFileName',{{'rti120xadc_c1_adc','OFF',[]}})  RTISFcnParameters=struct('ReadMode','int16','ChannelNo','int16','ConversionMode','int16','TriggerSource','int16','TriggerLineIn','int16','SampleMode','int16','BurstTriggerSource','int16','BurstTriggerLine','int16','ConvTriggerSource','int16','ConvTriggerLine','int16','ConvPeriod','double','BurstSize','int16','DataSetOffset','int16','DataSetLength','int16','EnableTriggerEvent','int16','TriggerMode','int16','TriggerLineOut','int16','ADCSWStartEnable','int16','SampleTime','double','StatusPortEnable','int16','TLCFileName','char')  RTIBlockParaDefault=struct('ReadMode',1,'ChannelNo',1,'ConversionMode',1,'TriggerSource',1,'TriggerLineIn',1,'SampleMode',1,'BurstTriggerSource',1,'BurstTriggerLine',1,'ConvTriggerSource',3,'ConvTriggerLine',1,'ConvPeriod',0.0001,'ConvPeriodCheck',0,'BurstSize',10,'BurstSizeCheck',0,'DataSetOffset',0,'DataSetOffsetCheck',0,'DataSetLength',1,'DataSetLengthCheck',0,'EnableTriggerEvent',0,'TriggerMode',2,'TriggerLineOut',1,'ADCSWStartEnable',0,'SampleTime',-1,'SampleTimeCheck',1,'StatusPortEnable',0,'TLCFileName','rti120xadc_c1_adc')
  Discrete Filter : DiscreteFilter  NumeratorSource=Input port  Numerator=[1-alpha]  DenominatorSource=Input port  Denominator=[1, alpha]  a0EqualsOne=on
      settings: InputPortMap=u0,p1,p3
  Divide : Product  Inputs=*/
  Divide1 : Product  Inputs=*/
  Divide2 : Product  Inputs=*/
  Subsystem : Subsystem
  acc_sns1 : Gain  Gain=1000/10.2
  alpha : Constant  Value=0.6
  amp1 : Constant
  amp2 : Constant
  amp3 : Constant
  disp_sns2 : Gain  Gain=7
  force_sns1 : Gain  Gain=1000/22.4
  in_gain1 : Gain  Gain=10
  in_gain2 : Gain  Gain=10
  in_gain3 : Gain  Gain=10
  Out1 : Outport
  Out2 : Outport  Port=2
  Out3 : Outport  Port=3
  wires:
  ADC_CLASS1_BL2/1 -> in_gain1/1
  Divide1/1 -> disp_sns2/1
  amp2/1 -> Divide1/2
  ADC_CLASS1_BL1/1 -> in_gain2/1
  in_gain2/1 -> Divide1/1
  in_gain1/1 -> Divide/1
  Divide/1 -> force_sns1/1
  amp1/1 -> Divide/2
  force_sns1/1 -> Out1/1
  disp_sns2/1 -> Discrete Filter/1
  in_gain3/1 -> Divide2/1
  acc_sns1/1 -> Out3/1
  amp3/1 -> Divide2/2
  ADC_CLASS1_BL3/1 -> in_gain3/1
  Divide2/1 -> acc_sns1/1
  Discrete Filter/1 -> Out2/1
  alpha/1 -> Subsystem/1(alpha)
  Subsystem/1(num) -> Discrete Filter/2
  Subsystem/2(den) -> Discrete Filter/3

== system sample_model/force_reconstructor ==
  coeffs : Inport
  fund_freq : Inport  Port=2
  Harmonic Basis Gen1 : Subsystem
  Product : Product
  Sum of Elements : Sum  Inputs=+
  Out1 : Outport
  wires:
  Product/1 -> Sum of Elements/1
  fund_freq/1 -> Harmonic Basis Gen1/1(fund_freq)
  Harmonic Basis Gen1/1(harmonic_basis) -> Product/2
  coeffs/1 -> Product/1
  Sum of Elements/1 -> Out1/1

== system sample_model/x_reconstructor ==
  coeffs : Inport
  fund_freq : Inport  Port=2
  Harmonic Basis Gen1 : Subsystem
  Product : Product
  Sum of Elements : Sum  Inputs=+
  Out1 : Outport
  wires:
  Sum of Elements/1 -> Out1/1
  coeffs/1 -> Product/1
  Harmonic Basis Gen1/1(harmonic_basis) -> Product/2
  fund_freq/1 -> Harmonic Basis Gen1/1(fund_freq)
  Product/1 -> Sum of Elements/1

== system sample_model/RTF_estimator/Subsystem ==
  input signal : Inport
  fund_freq : Inport  Port=2
  Fourier Series 2 : Subsystem
  Harmonic Basis Gen1 : Subsystem
  Fourier1 : Outport
  Phase1 : Outport  Port=2
  wires:
  Fourier Series 2/2(Phase) -> Phase1/1
  input signal/1 -> Fourier Series 2/1(input signal)
  Fourier Series 2/1(Fourier) -> Fourier1/1
  fund_freq/1 -> Harmonic Basis Gen1/1(fund_freq), Fourier Series 2/3(fundamental frequency)
  Harmonic Basis Gen1/1(harmonic_basis) -> Fourier Series 2/2(harmonic basis)

== system sample_model/RTF_estimator1/Subsystem ==
  input signal : Inport
  fund_freq : Inport  Port=2
  Fourier Series 2 : Subsystem
  Harmonic Basis Gen1 : Subsystem
  Fourier1 : Outport
  Phase1 : Outport  Port=2
  wires:
  Harmonic Basis Gen1/1(harmonic_basis) -> Fourier Series 2/2(harmonic basis)
  fund_freq/1 -> Fourier Series 2/3(fundamental frequency), Harmonic Basis Gen1/1(fund_freq)
  Fourier Series 2/1(Fourier) -> Fourier1/1
  input signal/1 -> Fourier Series 2/1(input signal)
  Fourier Series 2/2(Phase) -> Phase1/1

== system sample_model/RTI Data/RTI Data Store ==
  RTI Data Store : Subsystem  mask(RTI_DATA_STORE){}
      mask help:
      | RTI Data Store Block. This block is used by RTI to store internal model dependent data. Deleting this block will result in data loss.
      |
      | NEVER DELETE, COPY, OR MODIFY THIS BLOCK!
      mask Help:
      | RTI Data Store Block. This block is used by RTI to store internal model dependent data. Deleting this block will result in data loss.
      | 
      | NEVER DELETE, COPY, OR MODIFY THIS BLOCK!
      mask Display: text(0.5, 0.5, ' ', 'HorizontalAlignment', 'center');

== system sample_model/Transience_Estimator/get primary1 ==
  Vector : Inport
  Demux : Demux  Outputs=[1, 1, k_harmonics-1, 1, k_harmonics-1]
  Mux : Mux  Inputs=2
  Terminator2 : Terminator
  Terminator3 : Terminator
  Terminator4 : Terminator
  Primary : Outport
  wires:
  Vector/1 -> Demux/1
  Demux/5 -> Terminator4/1
  Demux/3 -> Terminator3/1
  Mux/1 -> Primary/1
  Demux/4 -> Mux/2
  Demux/2 -> Mux/1
  Demux/1 -> Terminator2/1

== system sample_model/Transience_Estimator/get primary4 ==
  Vector : Inport
  Demux : Demux  Outputs=[1, 1, k_harmonics-1, 1, k_harmonics-1]
  Mux : Mux  Inputs=2
  Terminator2 : Terminator
  Terminator3 : Terminator
  Terminator4 : Terminator
  Primary : Outport
  wires:
  Demux/1 -> Terminator2/1
  Demux/2 -> Mux/1
  Demux/4 -> Mux/2
  Mux/1 -> Primary/1
  Demux/3 -> Terminator3/1
  Demux/5 -> Terminator4/1
  Vector/1 -> Demux/1

== system sample_model/Transience_Estimator1/get primary1 ==
  Vector : Inport
  Demux : Demux  Outputs=[1, 1, k_harmonics-1, 1, k_harmonics-1]
  Mux : Mux  Inputs=2
  Terminator2 : Terminator
  Terminator3 : Terminator
  Terminator4 : Terminator
  Primary : Outport
  wires:
  Demux/1 -> Terminator2/1
  Demux/2 -> Mux/1
  Demux/4 -> Mux/2
  Mux/1 -> Primary/1
  Demux/3 -> Terminator3/1
  Demux/5 -> Terminator4/1
  Vector/1 -> Demux/1

== system sample_model/Transience_Estimator1/get primary4 ==
  Vector : Inport
  Demux : Demux  Outputs=[1, 1, k_harmonics-1, 1, k_harmonics-1]
  Mux : Mux  Inputs=2
  Terminator2 : Terminator
  Terminator3 : Terminator
  Terminator4 : Terminator
  Primary : Outport
  wires:
  Vector/1 -> Demux/1
  Demux/5 -> Terminator4/1
  Demux/3 -> Terminator3/1
  Mux/1 -> Primary/1
  Demux/4 -> Mux/2
  Demux/2 -> Mux/1
  Demux/1 -> Terminator2/1

== system sample_model/dSPACE in/Subsystem ==
  alpha : Inport
  Bias : Bias  Bias=1  SaturateOnIntegerOverflow=off
  Gain : Gain  Gain=-1
  num : Outport
  den : Outport  Port=2
  wires:
  Bias/1 -> num/1
  Gain/1 -> den/1, Bias/1
  alpha/1 -> Gain/1

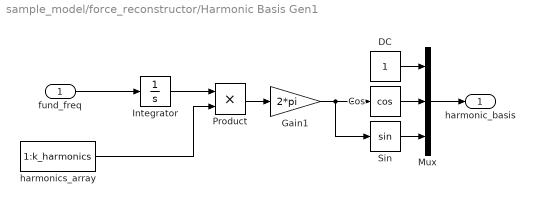
== system sample_model/force_reconstructor/Harmonic Basis Gen1 ==
  fund_freq : Inport
  Cos : Trigonometry  Operator=cos
  DC : Constant
  Gain1 : Gain  Gain=2*pi
  Integrator : Integrator
  Mux : Mux  Inputs=3
  Product : Product
  Sin : Trigonometry
  harmonics_array : Constant  Value=1:k_harmonics
  harmonic_basis : Outport  OutDataTypeStr=double  SampleTime=0
  wires:
  DC/1 -> Mux/1
  fund_freq/1 -> Integrator/1
  harmonics_array/1 -> Product/2
  Sin/1 -> Mux/3
  Product/1 -> Gain1/1
  Cos/1 -> Mux/2
  Integrator/1 -> Product/1
  Mux/1 -> harmonic_basis/1
  Gain1/1 -> Cos/1, Sin/1

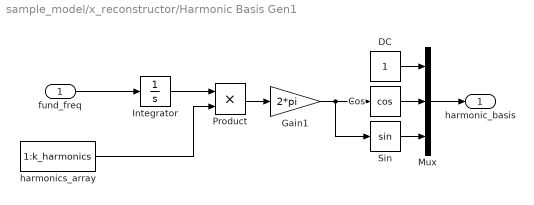
== system sample_model/x_reconstructor/Harmonic Basis Gen1 ==
  fund_freq : Inport
  Cos : Trigonometry  Operator=cos
  DC : Constant
  Gain1 : Gain  Gain=2*pi
  Integrator : Integrator
  Mux : Mux  Inputs=3
  Product : Product
  Sin : Trigonometry
  harmonics_array : Constant  Value=1:k_harmonics
  harmonic_basis : Outport  OutDataTypeStr=double  SampleTime=0
  wires:
  Gain1/1 -> Sin/1, Cos/1
  Mux/1 -> harmonic_basis/1
  Integrator/1 -> Product/1
  Cos/1 -> Mux/2
  Product/1 -> Gain1/1
  Sin/1 -> Mux/3
  harmonics_array/1 -> Product/2
  fund_freq/1 -> Integrator/1
  DC/1 -> Mux/1

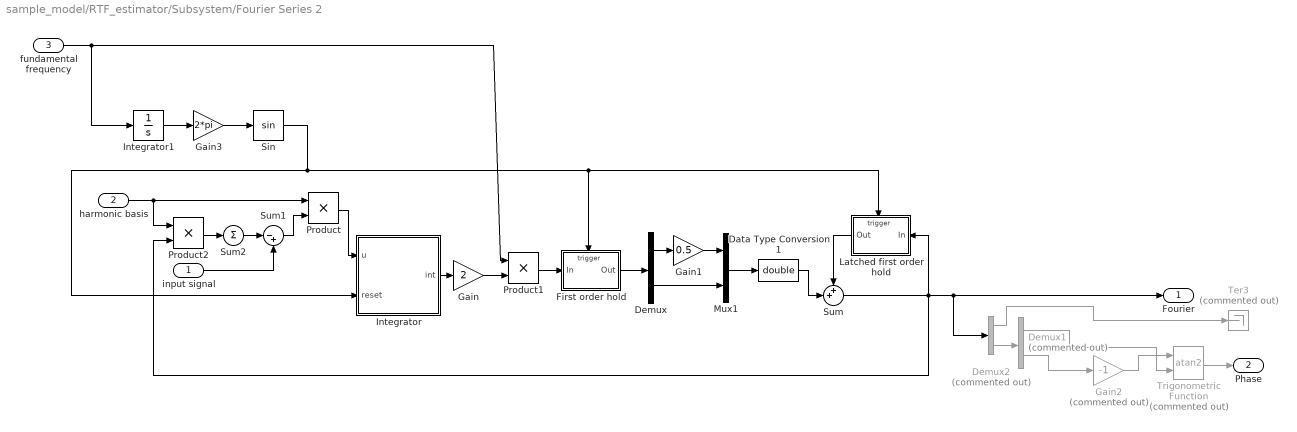
== system sample_model/RTF_estimator/Subsystem/Fourier Series 2 ==
  input signal : Inport
  harmonic basis : Inport  Port=2
  fundamental frequency : Inport  Port=3
  Data Type Conversion1 : DataTypeConversion  OutDataTypeStr=double  SaturateOnIntegerOverflow=off  RndMeth=Floor
  Demux : Demux  Outputs=[1 -1]
  Demux1 : Demux  Commented=on  Outputs=2
  Demux2 : Demux  Commented=on  Outputs=[1 -1]
  First order hold : Subsystem  TreatAsAtomicUnit=on
  Gain : Gain  Gain=2
  Gain1 : Gain  Gain=0.5
  Gain2 : Gain  Commented=on  Gain=-1
  Gain3 : Gain  Gain=2*pi
  Integrator : Subsystem
  Integrator1 : Integrator
  Latched first order hold : Subsystem  TreatAsAtomicUnit=on
  Mux1 : Mux  Inputs=2
  Product : Product  RndMeth=Zero
  Product1 : Product  RndMeth=Zero
  Product2 : Product  RndMeth=Zero
  Sin : Trigonometry
  Sum : Sum  Tag=Test  Inputs=++|
  Sum1 : Sum  Inputs=|-+
  Sum2 : Sum  Inputs=|+|
  Ter3 : Terminator  Commented=on
  Trigonometric Function : Trigonometry  Commented=on  Operator=atan2
  Fourier : Outport
  Phase : Outport  Port=2
  wires:
  fundamental frequency/1 -> Product1/1, Integrator1/1
  Integrator1/1 -> Gain3/1
  Gain3/1 -> Sin/1
  Demux2/1 -> Ter3/1
  Demux2/2 -> Demux1/1
  Gain2/1 -> Trigonometric Function/1
  Demux1/2 -> Gain2/1
  Demux1/1 -> Trigonometric Function/2
  Product/1 -> Integrator/1(u)
  Trigonometric Function/1 -> Phase/1
  Sum2/1 -> Sum1/1
  harmonic basis/1 -> Product2/1, Product/1
  input signal/1 -> Sum1/2
  Product2/1 -> Sum2/1
  Sum1/1 -> Product/2
  Latched first order hold/1(Out) -> Sum/1
  Sum/1 -> Demux2/1, Fourier/1, Latched first order hold/1(In), Product2/2
  Data Type Conversion1/1 -> Sum/2
  Mux1/1 -> Data Type Conversion1/1
  First order hold/1(Out) -> Demux/1
  Demux/2 -> Mux1/2
  Gain1/1 -> Mux1/1
  Demux/1 -> Gain1/1
  Integrator/1(int) -> Gain/1
  Sin/1 -> Latched first order hold/Trigger, First order hold/Trigger, Integrator/2(reset)
  Gain/1 -> Product1/2
  Product1/1 -> First order hold/1(In)

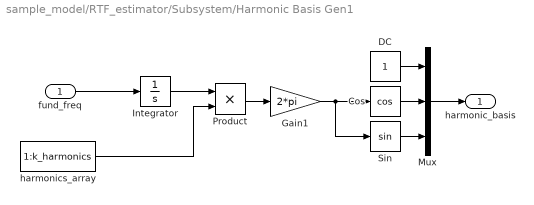
== system sample_model/RTF_estimator/Subsystem/Harmonic Basis Gen1 ==
  fund_freq : Inport
  Cos : Trigonometry  Operator=cos
  DC : Constant
  Gain1 : Gain  Gain=2*pi
  Integrator : Integrator
  Mux : Mux  Inputs=3
  Product : Product
  Sin : Trigonometry
  harmonics_array : Constant  Value=1:k_harmonics
  harmonic_basis : Outport  OutDataTypeStr=double  SampleTime=0
  wires:
  Gain1/1 -> Sin/1, Cos/1
  Mux/1 -> harmonic_basis/1
  Integrator/1 -> Product/1
  Cos/1 -> Mux/2
  Product/1 -> Gain1/1
  Sin/1 -> Mux/3
  harmonics_array/1 -> Product/2
  fund_freq/1 -> Integrator/1
  DC/1 -> Mux/1

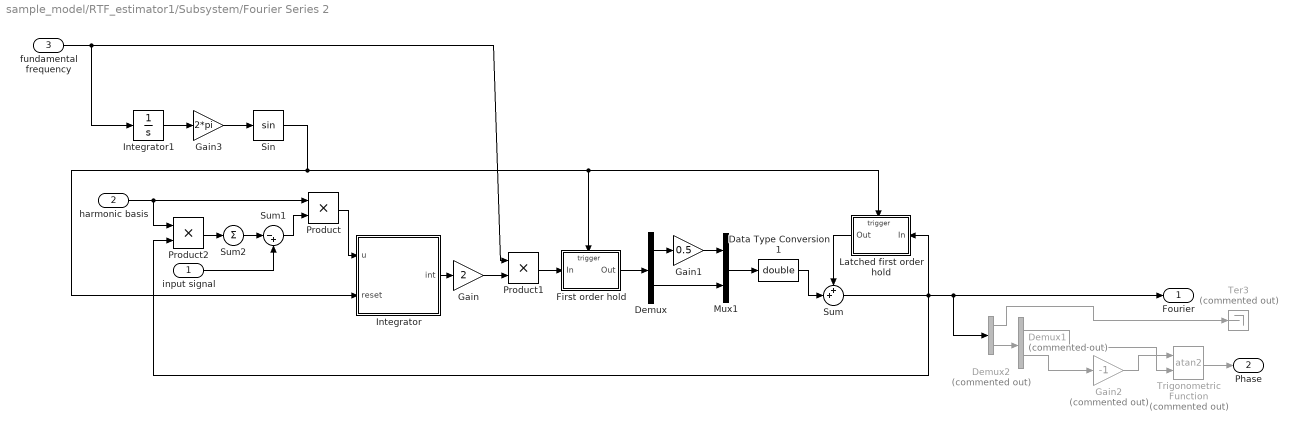
== system sample_model/RTF_estimator1/Subsystem/Fourier Series 2 ==
  input signal : Inport
  harmonic basis : Inport  Port=2
  fundamental frequency : Inport  Port=3
  Data Type Conversion1 : DataTypeConversion  OutDataTypeStr=double  SaturateOnIntegerOverflow=off  RndMeth=Floor
  Demux : Demux  Outputs=[1 -1]
  Demux1 : Demux  Commented=on  Outputs=2
  Demux2 : Demux  Commented=on  Outputs=[1 -1]
  First order hold : Subsystem  TreatAsAtomicUnit=on
  Gain : Gain  Gain=2
  Gain1 : Gain  Gain=0.5
  Gain2 : Gain  Commented=on  Gain=-1
  Gain3 : Gain  Gain=2*pi
  Integrator : Subsystem
  Integrator1 : Integrator
  Latched first order hold : Subsystem  TreatAsAtomicUnit=on
  Mux1 : Mux  Inputs=2
  Product : Product  RndMeth=Zero
  Product1 : Product  RndMeth=Zero
  Product2 : Product  RndMeth=Zero
  Sin : Trigonometry
  Sum : Sum  Tag=Test  Inputs=++|
  Sum1 : Sum  Inputs=|-+
  Sum2 : Sum  Inputs=|+|
  Ter3 : Terminator  Commented=on
  Trigonometric Function : Trigonometry  Commented=on  Operator=atan2
  Fourier : Outport
  Phase : Outport  Port=2
  wires:
  Product1/1 -> First order hold/1(In)
  Gain/1 -> Product1/2
  Sin/1 -> Integrator/2(reset), First order hold/Trigger, Latched first order hold/Trigger
  Integrator/1(int) -> Gain/1
  Demux/1 -> Gain1/1
  Gain1/1 -> Mux1/1
  Demux/2 -> Mux1/2
  First order hold/1(Out) -> Demux/1
  Mux1/1 -> Data Type Conversion1/1
  Data Type Conversion1/1 -> Sum/2
  Sum/1 -> Product2/2, Latched first order hold/1(In), Fourier/1, Demux2/1
  Latched first order hold/1(Out) -> Sum/1
  Sum1/1 -> Product/2
  Product2/1 -> Sum2/1
  input signal/1 -> Sum1/2
  harmonic basis/1 -> Product/1, Product2/1
  Sum2/1 -> Sum1/1
  Trigonometric Function/1 -> Phase/1
  Product/1 -> Integrator/1(u)
  Demux1/1 -> Trigonometric Function/2
  Demux1/2 -> Gain2/1
  Gain2/1 -> Trigonometric Function/1
  Demux2/2 -> Demux1/1
  Demux2/1 -> Ter3/1
  Gain3/1 -> Sin/1
  Integrator1/1 -> Gain3/1
  fundamental frequency/1 -> Integrator1/1, Product1/1

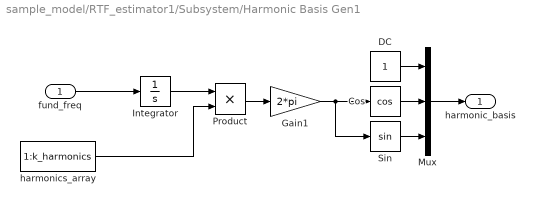
== system sample_model/RTF_estimator1/Subsystem/Harmonic Basis Gen1 ==
  fund_freq : Inport
  Cos : Trigonometry  Operator=cos
  DC : Constant
  Gain1 : Gain  Gain=2*pi
  Integrator : Integrator
  Mux : Mux  Inputs=3
  Product : Product
  Sin : Trigonometry
  harmonics_array : Constant  Value=1:k_harmonics
  harmonic_basis : Outport  OutDataTypeStr=double  SampleTime=0
  wires:
  DC/1 -> Mux/1
  fund_freq/1 -> Integrator/1
  harmonics_array/1 -> Product/2
  Sin/1 -> Mux/3
  Product/1 -> Gain1/1
  Cos/1 -> Mux/2
  Integrator/1 -> Product/1
  Mux/1 -> harmonic_basis/1
  Gain1/1 -> Cos/1, Sin/1

== system sample_model/RTI Data/RTI Data Store/RTI Data Store ==
  RTI Data Store : Subsystem  mask(RTI_DATA_STORE){}
      mask help:
      | RTI Data Store Block. This block is used by RTI to store internal model dependent data. Deleting this block will result in data loss.
      |
      | NEVER DELETE, COPY, OR MODIFY THIS BLOCK!
      mask Help:
      | RTI Data Store Block. This block is used by RTI to store internal model dependent data. Deleting this block will result in data loss.
      | 
      | NEVER DELETE, COPY, OR MODIFY THIS BLOCK!
      mask Display: text(0.5, 0.5, ' ', 'HorizontalAlignment', 'center');

== system sample_model/RTF_estimator/Subsystem/Fourier Series 2/First order hold ==
  In : Inport  LatchByDelayingOutsideSignal=on
  Trigger : TriggerPort  VariantControl=(inherit)
  Out : Outport
  wires:
  In/1 -> Out/1

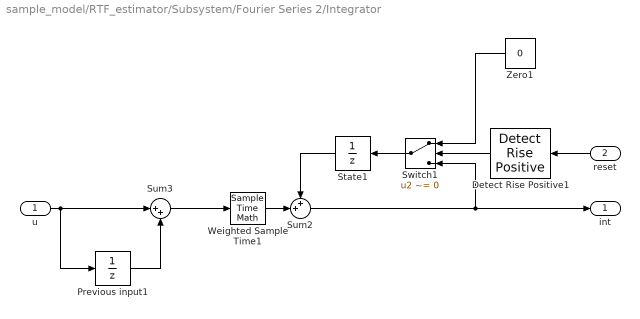
== system sample_model/RTF_estimator/Subsystem/Fourier Series 2/Integrator ==
  u : Inport
  reset : Inport  Port=2
  Detect Rise Positive1 : simulink/Logic and Bit Operations/Detect Rise Positive  vinit=0  OutDataTypeStr=uint8
  Previous input1 : UnitDelay  SampleTime=-1  HasFrameUpgradeWarning=on
  State1 : UnitDelay  SampleTime=-1  HasFrameUpgradeWarning=on
  Sum2 : Sum  Inputs=++|
  Sum3 : Sum  Inputs=|++
  Switch1 : Switch  Criteria=u2 ~= 0  SaturateOnIntegerOverflow=off  InputSameDT=off
  Weighted Sample Time1 : SampleTimeMath  TsampMathOp=*  weightValue=0.5
  Zero1 : Constant  Value=0
  int : Outport
  wires:
  State1/1 -> Sum2/1
  Sum2/1 -> Switch1/3, int/1
  Weighted Sample Time1/1 -> Sum2/2
  Sum3/1 -> Weighted Sample Time1/1
  u/1 -> Sum3/1, Previous input1/1
  Previous input1/1 -> Sum3/2
  reset/1 -> Detect Rise Positive1/1
  Switch1/1 -> State1/1
  Zero1/1 -> Switch1/1
  Detect Rise Positive1/1 -> Switch1/2

== system sample_model/RTF_estimator/Subsystem/Fourier Series 2/Latched first order hold ==
  In : Inport  LatchByDelayingOutsideSignal=on
  Trigger : TriggerPort  VariantControl=(inherit)
  Out : Outport
  wires:
  In/1 -> Out/1

== system sample_model/RTF_estimator1/Subsystem/Fourier Series 2/First order hold ==
  In : Inport  LatchByDelayingOutsideSignal=on
  Trigger : TriggerPort  VariantControl=(inherit)
  Out : Outport
  wires:
  In/1 -> Out/1
